simulink model "fuzzyPID"  (Simulink 7.0)
settings: Solver=ode3  StartTime=0.0  StopTime=50  MaxStep=0.01  MinStep=0.001  RelTol=1e-3
values from neighbouring files (symbols this model uses):
  dkd =     [fuzzpiddata.mat]
  dki =     [fuzzpiddata.mat]
  dkp =     [fuzzpiddata.mat]
settings Model: Creator=Administrator  LastModifiedBy=Administrator
settings OptimizationCC: InlineInvariantSignals=on
settings DebuggingCC: SaveWithParameterizedLinksMsg=none  SignalResolutionControl=TryResolveAllWithWarning  MultiTaskDSMMsg=warning  MultiTaskCondExecSysMsg=none  StrictBusMsg=None
settings RTWCC: IncludeERTFirstTime=on
settings GRTTargetCC: TargetFcnLib=ansi_tfl_tmw.mat

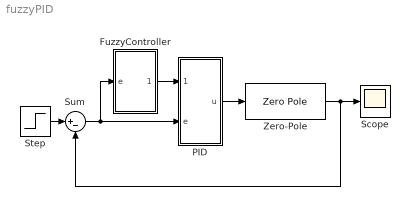
== system fuzzyPID ==
  FuzzyController : Subsystem
  PID : Subsystem
  Scope : Scope
      settings: TimeRange=50  YMin=0.5  YMax=1.1
  Step : Step  Time=0  SampleTime=0
  Sum : Sum  Inputs=|+-  OutDataType=sfix(16)  OutScaling=2^0
  Zero-Pole : ZeroPole  Zeros=[-0.5]  Poles=[-1 -1 -1]  Gain=[10]
  wires:
  Step/1 -> Sum/1
  Sum/1 -> PID/2(e), FuzzyController/1(e)
  PID/1(u) -> Zero-Pole/1
  Zero-Pole/1 -> Sum/2, Scope/1
  FuzzyController/1(dPID) -> PID/1(dPID)

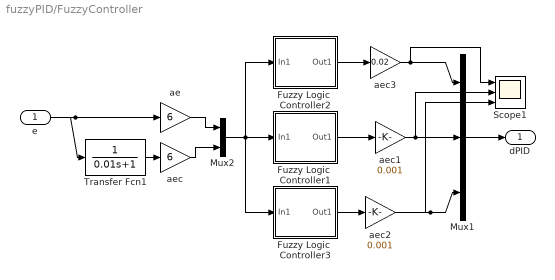
== system fuzzyPID/FuzzyController ==
  e : Inport  OutDataType=sfix(16)  OutScaling=2^0
  Fuzzy Logic  Controller1 : Subsystem  AncestorBlock="fuzblock/Fuzzy Logic  Controller"  mask(FIS){fis=dki}
      mask prompts: fis "FIS File or Structure:"
      mask help: FIS
      mask init:
      | fis = fuzblockmask(gcb,fis);
      mask Help: web(['file:///' docroot '/toolbox/fuzzy/fuzzylogiccontroller.html']);
      mask Display: plot(0, -0.3, 6, -0.3, 0, 1.2, 6, 1.2, [0 6], [0 0], [1 2 3],[0 1 0],[2 3 4],[0 1 0],[3 4 5],[0 1 0])
  Fuzzy Logic  Controller2 : Subsystem  AncestorBlock="fuzblock/Fuzzy Logic  Controller"  mask(FIS){fis=dkp}
      mask prompts: fis "FIS File or Structure:"
      mask help: FIS
      mask init:
      | fis = fuzblockmask(gcb,fis);
      mask Help: web(['file:///' docroot '/toolbox/fuzzy/fuzzylogiccontroller.html']);
      mask Display: plot(0, -0.3, 6, -0.3, 0, 1.2, 6, 1.2, [0 6], [0 0], [1 2 3],[0 1 0],[2 3 4],[0 1 0],[3 4 5],[0 1 0])
  Fuzzy Logic  Controller3 : Subsystem  AncestorBlock="fuzblock/Fuzzy Logic  Controller"  mask(FIS){fis=dkd}
      mask prompts: fis "FIS File or Structure:"
      mask help: FIS
      mask init:
      | fis = fuzblockmask(gcb,fis);
      mask Help: web(['file:///' docroot '/toolbox/fuzzy/fuzzylogiccontroller.html']);
      mask Display: plot(0, -0.3, 6, -0.3, 0, 1.2, 6, 1.2, [0 6], [0 0], [1 2 3],[0 1 0],[2 3 4],[0 1 0],[3 4 5],[0 1 0])
  Mux1 : Mux  Inputs=3
  Mux2 : Mux  Inputs=2
  Scope1 : Scope  NumInputPorts=3
      settings: TimeRange=10  YMin=0.975~-5~-5  YMax=1~5~5
  Transfer Fcn1 : TransferFcn  Denominator=[0.01 1]
  ae : Gain  Gain=6  ParameterDataType=sfix(16)  ParameterScaling=2^0  OutDataType=sfix(16)  OutScaling=2^0
  aec : Gain  Gain=6  ParameterDataType=sfix(16)  ParameterScaling=2^0  OutDataType=sfix(16)  OutScaling=2^0
  aec1 : Gain  Gain=0.001  ParameterDataType=sfix(16)  ParameterScaling=2^0  OutDataType=sfix(16)  OutScaling=2^0
  aec2 : Gain  Gain=0.001  ParameterDataType=sfix(16)  ParameterScaling=2^0  OutDataType=sfix(16)  OutScaling=2^0
  aec3 : Gain  Gain=0.02  ParameterDataType=sfix(16)  ParameterScaling=2^0  OutDataType=sfix(16)  OutScaling=2^0
  dPID : Outport
  wires:
  Fuzzy Logic  Controller2/1(Out1) -> aec3/1
  Fuzzy Logic  Controller1/1(Out1) -> aec1/1
  Fuzzy Logic  Controller3/1(Out1) -> aec2/1
  e/1 -> ae/1, Transfer Fcn1/1
  Transfer Fcn1/1 -> aec/1
  ae/1 -> Mux2/1
  aec/1 -> Mux2/2
  Mux2/1 -> Fuzzy Logic  Controller1/1(In1), Fuzzy Logic  Controller3/1(In1), Fuzzy Logic  Controller2/1(In1)
  aec1/1 -> Mux1/2, Scope1/2
  aec2/1 -> Mux1/3, Scope1/3
  aec3/1 -> Mux1/1, Scope1/1
  Mux1/1 -> dPID/1

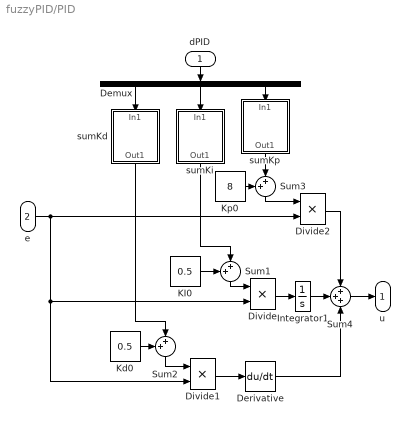
== system fuzzyPID/PID ==
  dPID : Inport  Orientation=down
  e : Inport  Port=2
  Demux : Demux  Orientation=down  Outputs=3
  Derivative : Derivative
  Divide : Product  Inputs=**  OutDataType=sfix(16)  OutScaling=2^-10
  Divide1 : Product  Inputs=**  OutDataType=sfix(16)  OutScaling=2^-10
  Divide2 : Product  Inputs=**  OutDataType=sfix(16)  OutScaling=2^-10
  Integrator1 : Integrator
  KI0 : Constant  Value=0.5  OutDataType=sfix(16)  OutScaling=2^0
  Kd0 : Constant  Value=0.5  OutDataType=sfix(16)  OutScaling=2^0
  Kp0 : Constant  Value=8  OutDataType=sfix(16)  OutScaling=2^0
  Sum1 : Sum  Orientation=down  Inputs=++|  OutDataType=sfix(16)  OutScaling=2^0
  Sum2 : Sum  Orientation=down  Inputs=++|  OutDataType=sfix(16)  OutScaling=2^0
  Sum3 : Sum  Orientation=down  Inputs=++|  OutDataType=sfix(16)  OutScaling=2^0
  Sum4 : Sum  Inputs=+++  OutDataType=sfix(16)  OutScaling=2^0
  sumKd : Subsystem  Orientation=down
  sumKi : Subsystem  Orientation=down
  sumKp : Subsystem  Orientation=down
  u : Outport  OutDataType=sfix(16)  OutScaling=2^0
  wires:
  Sum3/1 -> Divide2/1
  Sum2/1 -> Divide1/1
  Kp0/1 -> Sum3/1
  Kd0/1 -> Sum2/1
  KI0/1 -> Sum1/1
  Sum1/1 -> Divide/1
  e/1 -> Divide2/2, Divide/2, Divide1/2
  Divide2/1 -> Sum4/1
  Divide/1 -> Integrator1/1
  Divide1/1 -> Derivative/1
  Sum4/1 -> u/1
  dPID/1 -> Demux/1
  Demux/3 -> sumKp/1(In1)
  Demux/2 -> sumKi/1(In1)
  Demux/1 -> sumKd/1(In1)
  Integrator1/1 -> Sum4/2
  Derivative/1 -> Sum4/3
  sumKp/1(Out1) -> Sum3/2
  sumKi/1(Out1) -> Sum1/2
  sumKd/1(Out1) -> Sum2/2

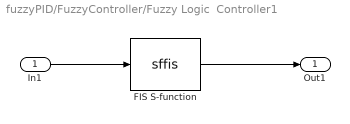
== system fuzzyPID/FuzzyController/Fuzzy Logic  Controller1 ==
  In1 : Inport  OutDataType=sfix(16)  OutScaling=2^0
  FIS S-function : S-Function  FunctionName=sffis  Parameters=fis  SFunctionModules=sfsup
  Out1 : Outport  OutDataType=sfix(16)  OutScaling=2^0
  wires:
  FIS S-function/1 -> Out1/1
  In1/1 -> FIS S-function/1

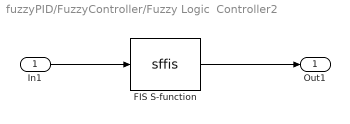
== system fuzzyPID/FuzzyController/Fuzzy Logic  Controller2 ==
  In1 : Inport  OutDataType=sfix(16)  OutScaling=2^0
  FIS S-function : S-Function  FunctionName=sffis  Parameters=fis  SFunctionModules=sfsup
  Out1 : Outport  OutDataType=sfix(16)  OutScaling=2^0
  wires:
  In1/1 -> FIS S-function/1
  FIS S-function/1 -> Out1/1

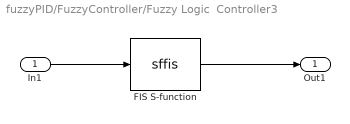
== system fuzzyPID/FuzzyController/Fuzzy Logic  Controller3 ==
  In1 : Inport  OutDataType=sfix(16)  OutScaling=2^0
  FIS S-function : S-Function  FunctionName=sffis  Parameters=fis  SFunctionModules=sfsup
  Out1 : Outport  OutDataType=sfix(16)  OutScaling=2^0
  wires:
  In1/1 -> FIS S-function/1
  FIS S-function/1 -> Out1/1

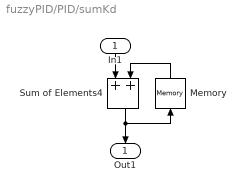
== system fuzzyPID/PID/sumKd ==
  In1 : Inport  Orientation=down
  Memory : Memory  Orientation=up  InheritSampleTime=on
  Sum of Elements4 : Sum  Orientation=down  OutDataType=sfix(16)  OutScaling=2^-10  SampleTime=0.001
  Out1 : Outport  Orientation=down
  wires:
  Sum of Elements4/1 -> Out1/1, Memory/1
  Memory/1 -> Sum of Elements4/2
  In1/1 -> Sum of Elements4/1

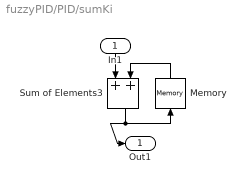
== system fuzzyPID/PID/sumKi ==
  In1 : Inport  Orientation=down
  Memory : Memory  Orientation=up  InheritSampleTime=on
  Sum of Elements3 : Sum  Orientation=down  OutDataType=sfix(16)  OutScaling=2^-10  SampleTime=0.001
  Out1 : Outport
  wires:
  Sum of Elements3/1 -> Out1/1, Memory/1
  Memory/1 -> Sum of Elements3/2
  In1/1 -> Sum of Elements3/1

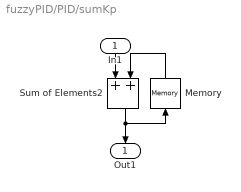
== system fuzzyPID/PID/sumKp ==
  In1 : Inport  Orientation=down
  Memory : Memory  Orientation=up  InheritSampleTime=on
  Sum of Elements2 : Sum  Orientation=down  OutDataType=sfix(16)  OutScaling=2^-10  SampleTime=0.001
  Out1 : Outport  Orientation=down
  wires:
  Sum of Elements2/1 -> Out1/1, Memory/1
  In1/1 -> Sum of Elements2/1
  Memory/1 -> Sum of Elements2/2
